simulink model "Model_IPS7"  (R2016a)
settings: Solver=FixedStepAuto  StartTime=0  StopTime=560  FixedStep=1e-5
InitFcn:
  | parametriAM
values from neighbouring files (symbols this model uses):
  Imrn = 7.4    [parametriAM.m]
  Ismax = In*sqrt(2)    [parametriAM.m]
  J = 0.019    [parametriAM.m]    (also in podatki.m = 0.01)
  Ki_Imr = 1000    [parametriAM.m]
  Ki_tok = 5.0    (= 5)    [parametriAM.m]
  Ki_wr = 1000    [parametriAM.m]
  Kp_Imr = 100    [parametriAM.m]
  Kp_tok = 0.05    [parametriAM.m]
  Kp_wr = 50    [parametriAM.m]
  Lm = 0.0493    [parametriAM.m]    (also in podatki.m = 0.2342)
  Lr = 0.05315    [parametriAM.m]    (also in podatki.m = 0.2449)
  Ls = 0.05315    [parametriAM.m]    (also in podatki.m = 0.2449)
  Lst = sigma*Ls    (= 0.00742111947319)    [parametriAM.m]
  naklon = naklon    [parametriAM.m]    (also in staticna_karakteristika.m = 1.0471975512)
  pp = 3    [parametriAM.m]    (also in podatki.m = 2)
  Rs = 0.594    [parametriAM.m]    (also in podatki.m = 3.7)
  sigma = 1 - 1/((1+sigmaR)*(1+sigmaS))    (= 0.13962595434)    [parametriAM.m]
  static_or_dinamic = static_or_dinamic    [parametriAM.m]    (also in potek_toka.m = 0; staticna_karakteristika.m = 5)
  Tr = Lr/Rr    (= 0.0771407837446)    [parametriAM.m]
  Udc = Un*sqrt(2)    [parametriAM.m]
  wb_upper_limit_field_weaking = sqrt((Ls^2+Lst^2)/(2*Lst^2*Ls^2))*Usmax/Ismax    [parametriAM.m]
  wdod = 2000*2*pi/60    (= 209.439510239)    [parametriAM.m]
  wn = Udc/sqrt(Ls^2*(Imrn)^2+Lst^2*(Ismax^2-(Imrn)^2))    [maximalnaelipsa.m]    (also in parametriAM.m = Un/sqrt(Ls^2*(Imrn)^2+Lst^2*(Ismax^2-(Imrn)^2))/pp)
libraries: simulink x25
(part 1 of 2)
settings Model: Creator=Vaje  LastModifiedBy=Mitja1

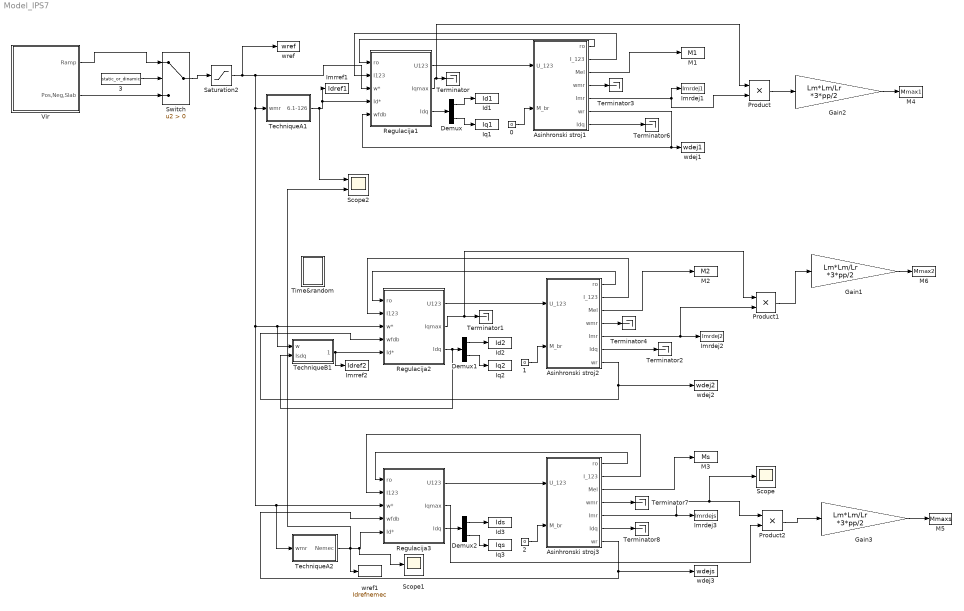
== system Model_IPS7 ==
  0 : Constant  Value=0
  1 : Constant  Value=0
  2 : Constant  Value=0
  3 : Constant  Value=static_or_dinamic
  Asinhronski stroj1 : Subsystem  InitFcn=parametriAM
  Asinhronski stroj2 : Subsystem  InitFcn=parametriAM
  Asinhronski stroj3 : Subsystem  InitFcn=parametriAM
  Demux : Demux  Outputs=2
  Demux1 : Demux  Outputs=2
  Demux2 : Demux  Outputs=2
  Gain1 : Gain  Gain=Lm*Lm/Lr *3*pp/2
  Gain2 : Gain  Gain=Lm*Lm/Lr *3*pp/2
  Gain3 : Gain  Gain=Lm*Lm/Lr *3*pp/2
  Id1 : ToWorkspace  VariableName=Id1  SampleTime=-1
      settings: Decimation=3  Save2DSignal=2-D array (concatenate along first dimension)
  Id2 : ToWorkspace  VariableName=Id2  SampleTime=-1
      settings: Decimation=3  Save2DSignal=2-D array (concatenate along first dimension)
  Id3 : ToWorkspace  VariableName=Ids  SampleTime=-1
      settings: Decimation=3  Save2DSignal=2-D array (concatenate along first dimension)
  Imrdej1 : ToWorkspace  VariableName=Imrdej1  SampleTime=-1
      settings: Decimation=3  Save2DSignal=2-D array (concatenate along first dimension)
  Imrdej2 : ToWorkspace  VariableName=Imrdej2  SampleTime=-1
      settings: Decimation=3  Save2DSignal=2-D array (concatenate along first dimension)
  Imrdej3 : ToWorkspace  VariableName=Imrdejs  SampleTime=-1
      settings: Decimation=3  Save2DSignal=2-D array (concatenate along first dimension)
  Imrref1 : ToWorkspace  VariableName=Idref1  SampleTime=-1
      settings: Decimation=3  Save2DSignal=2-D array (concatenate along first dimension)
  Imrref2 : ToWorkspace  VariableName=Idref2  SampleTime=-1
      settings: Decimation=3  Save2DSignal=2-D array (concatenate along first dimension)
  Iq1 : ToWorkspace  VariableName=Iq1  SampleTime=-1
      settings: Decimation=3  Save2DSignal=2-D array (concatenate along first dimension)
  Iq2 : ToWorkspace  VariableName=Iq2  SampleTime=-1
      settings: Decimation=3  Save2DSignal=2-D array (concatenate along first dimension)
  Iq3 : ToWorkspace  VariableName=Iqs  SampleTime=-1
      settings: Decimation=3  Save2DSignal=2-D array (concatenate along first dimension)
  M1 : ToWorkspace  VariableName=M1  SampleTime=-1
      settings: Decimation=3  Save2DSignal=2-D array (concatenate along first dimension)
  M2 : ToWorkspace  VariableName=M2  SampleTime=-1
      settings: Decimation=3  Save2DSignal=2-D array (concatenate along first dimension)
  M3 : ToWorkspace  VariableName=Ms  SampleTime=-1
      settings: Decimation=3  Save2DSignal=2-D array (concatenate along first dimension)
  M4 : ToWorkspace  VariableName=Mmax1  SampleTime=-1
      settings: Decimation=3  Save2DSignal=2-D array (concatenate along first dimension)
  M5 : ToWorkspace  VariableName=Mmaxs  SampleTime=-1
      settings: Decimation=3  Save2DSignal=2-D array (concatenate along first dimension)
  M6 : ToWorkspace  VariableName=Mmax2  SampleTime=-1
      settings: Decimation=3  Save2DSignal=2-D array (concatenate along first dimension)
  Product : Product
  Product1 : Product
  Product2 : Product
  Regulacija1 : Subsystem
  Regulacija2 : Subsystem
  Regulacija3 : Subsystem
  Saturation2 : Saturate  UpperLimit=wb_upper_limit_field_weaking  LowerLimit=-wb_upper_limit_field_weaking
  Scope : Scope
  Scope1 : Scope
  Scope2 : Scope  NumInputPorts=2
  Switch : Switch  Criteria=u2 > Threshold
  TechniqueA1 : Subsystem
  TechniqueA2 : Subsystem
  TechniqueB1 : Subsystem
  Terminator{,1..4,6..8} (8 alike) : Terminator
  Time&random : Subsystem
  Vir : Subsystem
  wdej1 : ToWorkspace  VariableName=wdej1  SampleTime=-1
      settings: Decimation=3  Save2DSignal=2-D array (concatenate along first dimension)
  wdej2 : ToWorkspace  VariableName=wdej2  SampleTime=-1
      settings: Decimation=3  Save2DSignal=2-D array (concatenate along first dimension)
  wdej3 : ToWorkspace  VariableName=wdejs  SampleTime=-1
      settings: Decimation=3  Save2DSignal=2-D array (concatenate along first dimension)
  wref : ToWorkspace  VariableName=wref  SampleTime=-1
      settings: Decimation=3  Save2DSignal=2-D array (concatenate along first dimension)
  wref1 : ToWorkspace  VariableName=Idrefnemec  SampleTime=-1
      settings: Decimation=3  Save2DSignal=2-D array (concatenate along first dimension)
  wires:
  Vir/2(Pos,Neg,Slab) -> Switch/3
  TechniqueA1/1(6.1-126) -> Scope2/1, Regulacija1/4(Id*), Imrref1/1
  Asinhronski stroj1/1(ro) -> Regulacija1/1(ro)
  Asinhronski stroj1/2(I_123) -> Regulacija1/2(I123)
  Regulacija1/1(U123) -> Asinhronski stroj1/1(U_123)
  Asinhronski stroj1/6(wr) -> Regulacija1/5(wfdb), wdej1/1
  Switch/1 -> Saturation2/1
  Asinhronski stroj2/1(ro) -> Regulacija2/1(ro)
  Asinhronski stroj2/2(I_123) -> Regulacija2/2(I123)
  Regulacija2/1(U123) -> Asinhronski stroj2/1(U_123)
  Saturation2/1 -> Regulacija1/3(w*), TechniqueA1/1(wmr), TechniqueA2/1(wmr), Regulacija3/3(w*), TechniqueB1/1(w), Regulacija2/3(w*), wref/1
  Regulacija2/3(Idq) -> TechniqueB1/2(Isdq), Demux1/1
  TechniqueB1/1(6.1-135) -> Regulacija2/5(Id*), Imrref2/1
  Asinhronski stroj1/5(Imr) -> Product/2, Imrdej1/1
  Asinhronski stroj2/5(Imr) -> Product1/2, Imrdej2/1
  Asinhronski stroj1/3(Mel) -> M1/1
  Asinhronski stroj2/3(Mel) -> M2/1
  Demux/2 -> Iq1/1
  Demux/1 -> Id1/1
  Demux1/1 -> Id2/1
  Demux1/2 -> Iq2/1
  Regulacija1/3(Idq) -> Demux/1
  Regulacija1/2(Iqmax) -> Product/1, Terminator/1
  Regulacija2/2(Iqmax) -> Product1/1, Terminator1/1
  Asinhronski stroj2/6(Idq) -> Terminator2/1
  0/1 -> Asinhronski stroj1/2(M_br)
  1/1 -> Asinhronski stroj2/2(M_br)
  Asinhronski stroj1/7(Idq) -> Terminator6/1
  Asinhronski stroj1/4(wmr) -> Terminator3/1
  Asinhronski stroj2/4(wmr) -> Terminator4/1
  Regulacija3/1(U123) -> Asinhronski stroj3/1(U_123)
  Regulacija3/3(Idq) -> Demux2/1
  Demux2/1 -> Id3/1
  Demux2/2 -> Iq3/1
  Regulacija3/2(Iqmax) -> Product2/2
  2/1 -> Asinhronski stroj3/2(M_br)
  Asinhronski stroj3/1(ro) -> Regulacija3/1(ro)
  Asinhronski stroj3/2(I_123) -> Regulacija3/2(I123)
  Asinhronski stroj3/5(Imr) -> Scope/1, Product2/1, Imrdej3/1
  Asinhronski stroj3/3(Mel) -> M3/1
  Asinhronski stroj3/4(wmr) -> Terminator7/1
  Asinhronski stroj3/6(Idq) -> Terminator8/1
  Product/1 -> Gain2/1
  Product1/1 -> Gain1/1
  Product2/1 -> Gain3/1
  Gain2/1 -> M4/1
  Gain3/1 -> M5/1
  Gain1/1 -> M6/1
  3/1 -> Switch/2
  Asinhronski stroj3/7(wr) -> wdej3/1, Regulacija3/4(wfdb)
  Asinhronski stroj2/7(wr) -> Regulacija2/4(wfdb), wdej2/1
  Vir/1(Ramp) -> Switch/1
  TechniqueA2/1(Nemec) -> Scope2/2, wref1/1, Scope1/1, Regulacija3/5(Id*)

== system Model_IPS7/Asinhronski stroj1 ==
  U_123 : Inport
  M_br : Inport  Port=2
  Clarke : Subsystem
  Inverzni Clarke : Subsystem
  Inverzni Park : Subsystem
  Mehanika : Subsystem
  Park : Subsystem
  napetostni dq model : Subsystem
  ro : Outport
  I_123 : Outport  Port=2
  Mel : Outport  Port=3
  wmr : Outport  Port=4
  Imr : Outport  Port=5
  wr : Outport  Port=6
  Idq : Outport  Port=7
  wires:
  Inverzni Park/1(I_ab) -> Inverzni Clarke/1(I_ab)
  Clarke/1(U_ab) -> Park/1(U_ab)
  Mehanika/1(wr) -> napetostni dq model/2(wr), wr/1
  M_br/1 -> Mehanika/1(M_br)
  napetostni dq model/1(Mel) -> Mel/1, Mehanika/2(M_el)
  Inverzni Clarke/1(I_123) -> I_123/1
  napetostni dq model/4(wmr) -> wmr/1
  napetostni dq model/3(Imr) -> Imr/1
  U_123/1 -> Clarke/1(U_123)
  napetostni dq model/2(Is_dq) -> Idq/1, Inverzni Park/1(I_dq)
  napetostni dq model/5(ro) -> ro/1, Park/2(kot), Inverzni Park/2(kot)
  Park/1(U_dq) -> napetostni dq model/1(Us_dq)

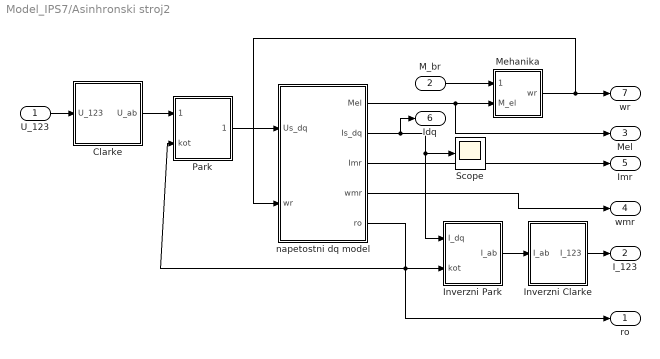
== system Model_IPS7/Asinhronski stroj2 ==
  U_123 : Inport
  M_br : Inport  Port=2
  Clarke : Subsystem
  Inverzni Clarke : Subsystem
  Inverzni Park : Subsystem
  Mehanika : Subsystem
  Park : Subsystem
  Scope : Scope
  napetostni dq model : Subsystem
  ro : Outport
  I_123 : Outport  Port=2
  Mel : Outport  Port=3
  wmr : Outport  Port=4
  Imr : Outport  Port=5
  Idq : Outport  Port=6
  wr : Outport  Port=7
  wires:
  Inverzni Park/1(I_ab) -> Inverzni Clarke/1(I_ab)
  Clarke/1(U_ab) -> Park/1(U_ab)
  Mehanika/1(wr) -> napetostni dq model/2(wr), wr/1
  M_br/1 -> Mehanika/1(M_br)
  napetostni dq model/1(Mel) -> Mel/1, Mehanika/2(M_el)
  Inverzni Clarke/1(I_123) -> I_123/1
  napetostni dq model/4(wmr) -> wmr/1
  napetostni dq model/3(Imr) -> Imr/1
  U_123/1 -> Clarke/1(U_123)
  napetostni dq model/2(Is_dq) -> Idq/1, Scope/1, Inverzni Park/1(I_dq)
  napetostni dq model/5(ro) -> ro/1, Park/2(kot), Inverzni Park/2(kot)
  Park/1(U_dq) -> napetostni dq model/1(Us_dq)

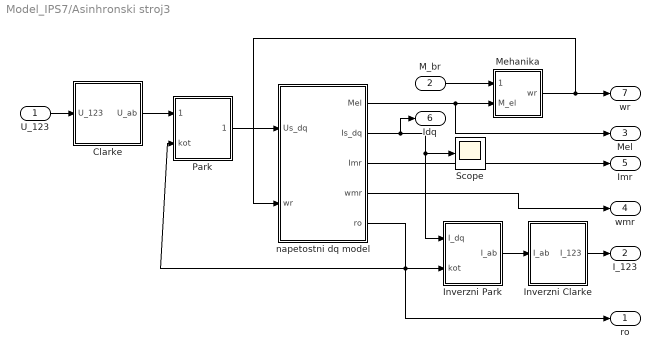
== system Model_IPS7/Asinhronski stroj3 ==
  U_123 : Inport
  M_br : Inport  Port=2
  Clarke : Subsystem
  Inverzni Clarke : Subsystem
  Inverzni Park : Subsystem
  Mehanika : Subsystem
  Park : Subsystem
  Scope : Scope
  napetostni dq model : Subsystem
  ro : Outport
  I_123 : Outport  Port=2
  Mel : Outport  Port=3
  wmr : Outport  Port=4
  Imr : Outport  Port=5
  Idq : Outport  Port=6
  wr : Outport  Port=7
  wires:
  Park/1(U_dq) -> napetostni dq model/1(Us_dq)
  napetostni dq model/5(ro) -> Inverzni Park/2(kot), Park/2(kot), ro/1
  napetostni dq model/2(Is_dq) -> Inverzni Park/1(I_dq), Scope/1, Idq/1
  U_123/1 -> Clarke/1(U_123)
  napetostni dq model/3(Imr) -> Imr/1
  napetostni dq model/4(wmr) -> wmr/1
  Inverzni Clarke/1(I_123) -> I_123/1
  napetostni dq model/1(Mel) -> Mehanika/2(M_el), Mel/1
  M_br/1 -> Mehanika/1(M_br)
  Mehanika/1(wr) -> wr/1, napetostni dq model/2(wr)
  Clarke/1(U_ab) -> Park/1(U_ab)
  Inverzni Park/1(I_ab) -> Inverzni Clarke/1(I_ab)

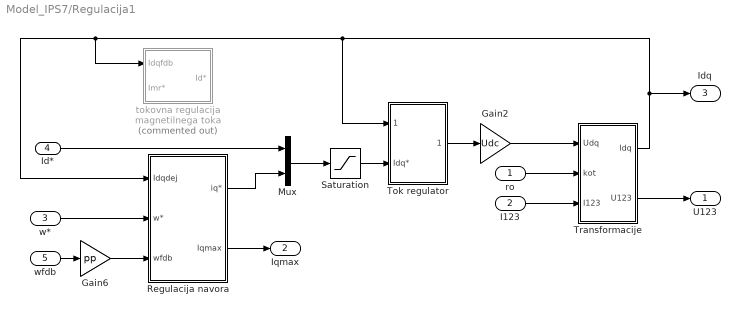
== system Model_IPS7/Regulacija1 ==
  ro : Inport
  I123 : Inport  Port=2
  w* : Inport  Port=3
  Id* : Inport  Port=4
  wfdb : Inport  Port=5
  Gain2 : Gain  Gain=Udc
  Gain6 : Gain  Gain=pp
  Mux : Mux  Inputs=2
  Regulacija navora : Subsystem
  Saturation : Saturate  UpperLimit=Ismax  LowerLimit=-Ismax
  Tok regulator : Subsystem
  Transformacije : Subsystem
  tokovna regulacija magnetilnega toka : Subsystem  Commented=on
  U123 : Outport
  Iqmax : Outport  Port=2
  Idq : Outport  Port=3
  wires:
  w*/1 -> Regulacija navora/2(w*)
  Transformacije/1(Idq) -> Idq/1, Tok regulator/1(Idqdej), tokovna regulacija magnetilnega toka/1(Idqfdb), Regulacija navora/1(Idqdej)
  ro/1 -> Transformacije/2(kot)
  I123/1 -> Transformacije/3(I123)
  Gain2/1 -> Transformacije/1(Udq)
  wfdb/1 -> Gain6/1
  Mux/1 -> Saturation/1
  Tok regulator/1(Udq*) -> Gain2/1
  Regulacija navora/1(iq*) -> Mux/2
  Transformacije/2(U123) -> U123/1
  Regulacija navora/2(Iqmax) -> Iqmax/1
  Gain6/1 -> Regulacija navora/3(wfdb)
  Saturation/1 -> Tok regulator/2(Idq*)
  Id*/1 -> Mux/1

== system Model_IPS7/Regulacija2 ==
  ro : Inport
  I123 : Inport  Port=2
  w* : Inport  Port=3
  wfdb : Inport  Port=4
  Id* : Inport  Port=5
  Gain2 : Gain  Gain=Udc
  Gain6 : Gain  Gain=pp
  Mux : Mux  Inputs=2
  Regulacija navora : Subsystem
  Tok regulator : Subsystem
  Transformacije : Subsystem
  tokovna regulacija magnetilnega toka : Subsystem  Commented=on
  U123 : Outport
  Iqmax : Outport  Port=2
  Idq : Outport  Port=3
  wires:
  Id*/1 -> Mux/1
  w*/1 -> Regulacija navora/2(w*)
  Transformacije/1(Idq) -> Tok regulator/1(Idqdej), Regulacija navora/1(Idqdej), tokovna regulacija magnetilnega toka/1(Idqfdb), Idq/1
  ro/1 -> Transformacije/2(kot)
  I123/1 -> Transformacije/3(I123)
  Gain2/1 -> Transformacije/1(Udq)
  wfdb/1 -> Gain6/1
  Mux/1 -> Tok regulator/2(Idq*)
  Tok regulator/1(Udq*) -> Gain2/1
  Regulacija navora/1(Iq*) -> Mux/2
  Transformacije/2(U123) -> U123/1
  Regulacija navora/2(Iqmax) -> Iqmax/1
  Gain6/1 -> Regulacija navora/3(wfdb)

== system Model_IPS7/Regulacija3 ==
  ro : Inport
  I123 : Inport  Port=2
  w* : Inport  Port=3
  wfdb : Inport  Port=4
  Id* : Inport  Port=5
  Gain2 : Gain  Gain=Udc
  Gain6 : Gain  Gain=pp
  Mux : Mux  Inputs=2
  Regulacija navora : Subsystem
  Tok regulator : Subsystem
  Transformacije : Subsystem
  tokovna regulacija magnetilnega toka : Subsystem
  U123 : Outport
  Iqmax : Outport  Port=2
  Idq : Outport  Port=3
  wires:
  Gain6/1 -> Regulacija navora/3(wfdb)
  Regulacija navora/2(Iqmax) -> Iqmax/1
  Transformacije/2(U123) -> U123/1
  Regulacija navora/1(Iq*) -> Mux/2
  Tok regulator/1(Udq*) -> Gain2/1
  Mux/1 -> Tok regulator/2(Idq*)
  wfdb/1 -> Gain6/1
  Gain2/1 -> Transformacije/1(Udq)
  I123/1 -> Transformacije/3(I123)
  ro/1 -> Transformacije/2(kot)
  Transformacije/1(Idq) -> Idq/1, tokovna regulacija magnetilnega toka/1(Idqfdb), Regulacija navora/1(Idqdej), Tok regulator/1(Idqdej)
  w*/1 -> Regulacija navora/2(w*)
  tokovna regulacija magnetilnega toka/1(Id*) -> Mux/1
  Id*/1 -> tokovna regulacija magnetilnega toka/2(Imr*)

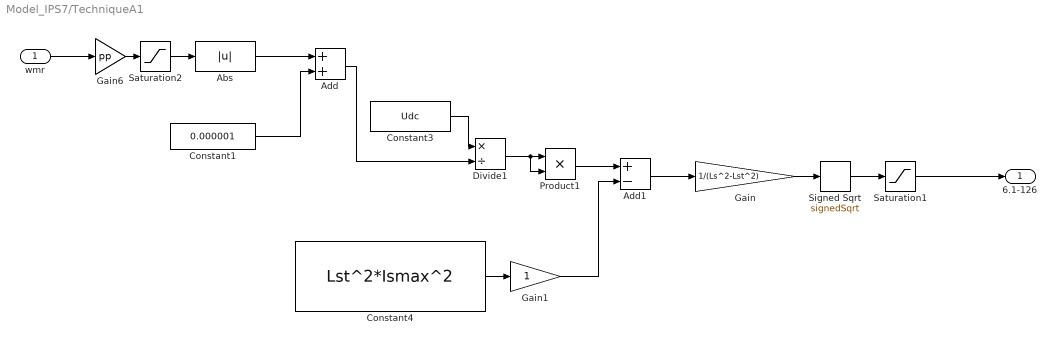
== system Model_IPS7/TechniqueA1 ==
  wmr : Inport
  Abs : Abs
  Add : Sum
  Add1 : Sum  Inputs=+-
  Constant1 : Constant  Value=0.000001
  Constant3 : Constant  Value=Udc
  Constant4 : Constant  Value=Lst^2*Ismax^2
  Divide1 : Product  Inputs=*/
  Gain : Gain  Gain=1/(Ls^2-Lst^2)
  Gain1 : Gain
  Gain6 : Gain  Gain=pp
  Product1 : Product
  Saturation1 : Saturate  UpperLimit=+Imrn*sqrt(2)  LowerLimit=-Imrn*sqrt(2)
  Saturation2 : Saturate  UpperLimit=wb_upper_limit_field_weaking  LowerLimit=-wb_upper_limit_field_weaking
  Signed Sqrt : Sqrt  Operator=signedSqrt  SaturateOnIntegerOverflow=on
  6.1-126 : Outport
  wires:
  Add/1 -> Divide1/2
  Abs/1 -> Add/1
  Constant1/1 -> Add/2
  Constant3/1 -> Divide1/1
  Divide1/1 -> Product1/2, Product1/1
  Product1/1 -> Add1/1
  Saturation1/1 -> 6.1-126/1
  Add1/1 -> Gain/1
  Gain/1 -> Signed Sqrt/1
  Signed Sqrt/1 -> Saturation1/1
  Saturation2/1 -> Abs/1
  Constant4/1 -> Gain1/1
  Gain1/1 -> Add1/2
  Gain6/1 -> Saturation2/1
  wmr/1 -> Gain6/1

== system Model_IPS7/TechniqueA2 ==
  wmr : Inport
  Abs : Abs
  Add : Sum
  Constant : Constant  Value=wn
  Constant1 : Constant  Value=0.000001
  Constant2 : Constant  Value=Imrn*sqrt(2)
  Divide : Product  Inputs=*/
  Product : Product
  Saturation : Saturate  UpperLimit=+Imrn*sqrt(2)  LowerLimit=-Imrn*sqrt(2)
  Saturation2 : Saturate  UpperLimit=wb_upper_limit_field_weaking  LowerLimit=-wb_upper_limit_field_weaking
  Nemec : Outport
  wires:
  Saturation2/1 -> Abs/1
  Saturation/1 -> Nemec/1
  Constant1/1 -> Add/2
  Abs/1 -> Add/1
  Add/1 -> Divide/2
  Constant/1 -> Divide/1
  Product/1 -> Saturation/1
  Divide/1 -> Product/2
  Constant2/1 -> Product/1
  wmr/1 -> Saturation2/1

== system Model_IPS7/TechniqueB1 ==
  w : Inport
  Isdq : Inport  Port=2
  Add4 : Sum
  Const c : Subsystem
  Deljeno imenovalec 6.1-135 : Gain  Gain=1/(Ls^2-Lst^2)
  Demux : Demux  Outputs=2
  Gain4 : Gain  Gain=-Ls
  Gain6 : Gain  Gain=pp
  Korenski del : Subsystem
  Saturation : Saturate  UpperLimit=+Imrn*sqrt(2)  LowerLimit=-Imrn*sqrt(2)
  Terminator : Terminator
  6.1-135 : Outport
  wires:
  Demux/1 -> Const c/1(Id)
  Demux/2 -> Terminator/1
  Saturation/1 -> 6.1-135/1
  Const c/1(c) -> Korenski del/1(c), Gain4/1
  Gain4/1 -> Add4/1
  Add4/1 -> Deljeno imenovalec 6.1-135/1
  Deljeno imenovalec 6.1-135/1 -> Saturation/1
  Isdq/1 -> Demux/1
  Korenski del/1(korenjen del) -> Add4/2
  w/1 -> Gain6/1
  Gain6/1 -> Korenski del/2(w)

== system Model_IPS7/Time&random ==
  99% max navora : Subsystem  Commented=on
  Mux1 : Mux  Commented=on  Inputs=2
  Ramp : simulink/Sources/Ramp  slope=1  start=0  X0=0
  To Workspace3 : ToWorkspace  VariableName=time  SampleTime=-1
      settings: Decimation=3  Save2DSignal=2-D array (concatenate along first dimension)
  wires:
  Ramp/1 -> To Workspace3/1

== system Model_IPS7/Vir ==
  Add1 : Sum
  Rampa : simulink/Sources/Ramp  slope=naklon  start=0.3  X0=0
  Step : Step  Time=0.1  After=2000*2*pi/60  SampleTime=0
  Step1 : Step  Time=0.7  After=2000*pi/30  SampleTime=0
  Step2 : Step  Commented=on  Time=2  After=2000*2*pi/60  SampleTime=0
  Step3 : Step  Commented=on  Time=3  After=2000*2*pi/60  SampleTime=0
  Step4 : Step  Commented=on  Time=8  After=wdod  SampleTime=0
  Step5 : Step  Commented=on  Time=9  After=wdod  SampleTime=0
  Ramp : Outport
  Pos,Neg,Slab : Outport  Port=2
  wires:
  Add1/1 -> Pos,Neg,Slab/1
  Step/1 -> Add1/1
  Rampa/1 -> Ramp/1
  Step1/1 -> Add1/2

== system Model_IPS7/Asinhronski stroj1/Clarke ==
  U_123 : Inport
  ABC_ab1 : Subsystem
  Demux : Demux  Outputs=3
  Mux : Mux  Inputs=2
  U_ab : Outport
  wires:
  Mux/1 -> U_ab/1
  ABC_ab1/2(beta) -> Mux/2
  ABC_ab1/1(alfa) -> Mux/1
  Demux/3 -> ABC_ab1/3(C)
  Demux/2 -> ABC_ab1/2(B)
  Demux/1 -> ABC_ab1/1(A)
  U_123/1 -> Demux/1

== system Model_IPS7/Asinhronski stroj1/Inverzni Clarke ==
  I_ab : Inport
  Demux : Demux  Outputs=2
  Mux : Mux  Inputs=3
  ab_ABC : Subsystem
  I_123 : Outport
  wires:
  ab_ABC/3(C) -> Mux/3
  ab_ABC/2(B) -> Mux/2
  ab_ABC/1(A) -> Mux/1
  Demux/2 -> ab_ABC/2(beta)
  Demux/1 -> ab_ABC/1(alfa)
  I_ab/1 -> Demux/1
  Mux/1 -> I_123/1

== system Model_IPS7/Asinhronski stroj1/Inverzni Park ==
  I_dq : Inport
  kot : Inport  Port=2
  Demux : Demux  Outputs=2
  Mux : Mux  Inputs=2
  "Sum1 " : Sum  Inputs=+-  SaturateOnIntegerOverflow=on  InputSameDT=on  OutDataTypeStr=Inherit: Same as first input
  Sum2 : Sum  SaturateOnIntegerOverflow=on  InputSameDT=on  OutDataTypeStr=Inherit: Same as first input
  cos : Fcn  Expr=cos(u)
  sin : Fcn  Expr=sin(u)
  x_d*cos : Product  SaturateOnIntegerOverflow=on  RndMeth=Zero  InputSameDT=on  OutDataTypeStr=Inherit: Same as first input
  x_d*sin : Product  SaturateOnIntegerOverflow=on  RndMeth=Zero  InputSameDT=on  OutDataTypeStr=Inherit: Same as first input
  x_q*cos : Product  SaturateOnIntegerOverflow=on  RndMeth=Zero  InputSameDT=on  OutDataTypeStr=Inherit: Same as first input
  "x_q*sin " : Product  SaturateOnIntegerOverflow=on  RndMeth=Zero  InputSameDT=on  OutDataTypeStr=Inherit: Same as first input
  I_ab : Outport
  wires:
  Mux/1 -> I_ab/1
  I_dq/1 -> Demux/1
  Demux/1 -> x_d*sin/1, x_d*cos/1
  Demux/2 -> "x_q*sin "/1, x_q*cos/1
  cos/1 -> x_q*cos/2, x_d*cos/2
  sin/1 -> "x_q*sin "/2, x_d*sin/2
  x_d*cos/1 -> "Sum1 "/1
  "x_q*sin "/1 -> "Sum1 "/2
  x_q*cos/1 -> Sum2/2
  x_d*sin/1 -> Sum2/1
  "Sum1 "/1 -> Mux/1
  Sum2/1 -> Mux/2
  kot/1 -> cos/1, sin/1

== system Model_IPS7/Asinhronski stroj1/Mehanika ==
  M_br : Inport
  M_el : Inport  Port=2
  Sum : Sum  Inputs=+-
  eq 2.19 : Subsystem
  wr : Outport
  wires:
  M_br/1 -> Sum/2
  Sum/1 -> eq 2.19/1(M)
  M_el/1 -> Sum/1
  eq 2.19/1(wr) -> wr/1

== system Model_IPS7/Asinhronski stroj1/Park ==
  U_ab : Inport
  kot : Inport  Port=2
  Demux : Demux  Outputs=2
  Mux : Mux  Inputs=2
  "Sum1 " : Sum  SaturateOnIntegerOverflow=on  InputSameDT=on  OutDataTypeStr=Inherit: Same as first input
  Sum2 : Sum  Inputs=-+  SaturateOnIntegerOverflow=on  InputSameDT=on  OutDataTypeStr=Inherit: Same as first input
  cos : Fcn  Expr=cos(u)
  sin : Fcn  Expr=sin(u)
  x_a*cos : Product  SaturateOnIntegerOverflow=on  RndMeth=Zero  InputSameDT=on  OutDataTypeStr=Inherit: Same as first input
  x_a*sin : Product  SaturateOnIntegerOverflow=on  RndMeth=Zero  InputSameDT=on  OutDataTypeStr=Inherit: Same as first input
  x_b*cos : Product  SaturateOnIntegerOverflow=on  RndMeth=Zero  InputSameDT=on  OutDataTypeStr=Inherit: Same as first input
  "x_b*sin " : Product  SaturateOnIntegerOverflow=on  RndMeth=Zero  InputSameDT=on  OutDataTypeStr=Inherit: Same as first input
  U_dq : Outport
  wires:
  Mux/1 -> U_dq/1
  U_ab/1 -> Demux/1
  Demux/1 -> x_a*sin/1, x_a*cos/1
  Demux/2 -> "x_b*sin "/1, x_b*cos/1
  cos/1 -> x_b*cos/2, x_a*cos/2
  sin/1 -> "x_b*sin "/2, x_a*sin/2
  x_a*cos/1 -> "Sum1 "/1
  "x_b*sin "/1 -> "Sum1 "/2
  x_b*cos/1 -> Sum2/2
  x_a*sin/1 -> Sum2/1
  "Sum1 "/1 -> Mux/1
  Sum2/1 -> Mux/2
  kot/1 -> cos/1, sin/1

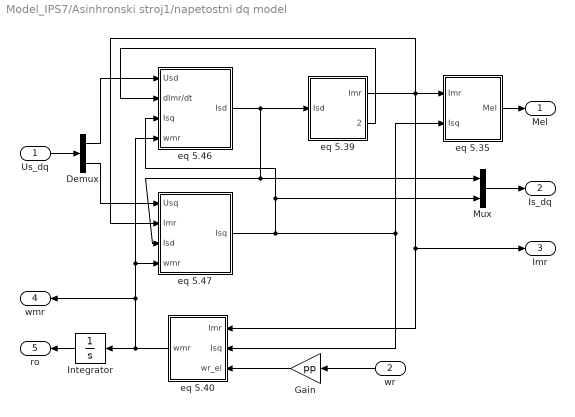
== system Model_IPS7/Asinhronski stroj1/napetostni dq model ==
  Us_dq : Inport
  wr : Inport  Port=2
  Demux : Demux  Outputs=2
  Gain : Gain  Gain=pp
  Integrator : Integrator
  Mux : Mux  Inputs=2
  eq 5.35 : Subsystem
  eq 5.39 : Subsystem
  eq 5.40 : Subsystem
  eq 5.46 : Subsystem
  eq 5.47 : Subsystem
  Mel : Outport
  Is_dq : Outport  Port=2
  Imr : Outport  Port=3
  wmr : Outport  Port=4
  ro : Outport  Port=5
  wires:
  Gain/1 -> eq 5.40/3(wr_el)
  Mux/1 -> Is_dq/1
  Demux/2 -> eq 5.47/1(Usq)
  Demux/1 -> eq 5.46/1(Usd)
  Us_dq/1 -> Demux/1
  wr/1 -> Gain/1
  Integrator/1 -> ro/1
  eq 5.35/1(Mel) -> Mel/1
  eq 5.40/1(wmr) -> Integrator/1, wmr/1, eq 5.46/4(wmr), eq 5.47/4(wmr)
  eq 5.47/1(Isq) -> Mux/2, eq 5.46/3(Isq), eq 5.40/2(Isq), eq 5.35/2(Isq)
  eq 5.39/1(Imr) -> eq 5.47/2(Imr), Imr/1, eq 5.40/1(Imr), eq 5.35/1(Imr)
  eq 5.39/2(dImr/dt) -> eq 5.46/2(dImr/dt)
  eq 5.46/1(Isd) -> Mux/1, eq 5.47/3(Isd), eq 5.39/1(Isd)

== system Model_IPS7/Asinhronski stroj2/Clarke ==
  U_123 : Inport
  ABC_ab1 : Subsystem
  Demux : Demux  Outputs=3
  Mux : Mux  Inputs=2
  U_ab : Outport
  wires:
  Mux/1 -> U_ab/1
  ABC_ab1/2(beta) -> Mux/2
  ABC_ab1/1(alfa) -> Mux/1
  Demux/3 -> ABC_ab1/3(C)
  Demux/2 -> ABC_ab1/2(B)
  Demux/1 -> ABC_ab1/1(A)
  U_123/1 -> Demux/1

== system Model_IPS7/Asinhronski stroj2/Inverzni Clarke ==
  I_ab : Inport
  Demux : Demux  Outputs=2
  Mux : Mux  Inputs=3
  ab_ABC : Subsystem
  I_123 : Outport
  wires:
  ab_ABC/3(C) -> Mux/3
  ab_ABC/2(B) -> Mux/2
  ab_ABC/1(A) -> Mux/1
  Demux/2 -> ab_ABC/2(beta)
  Demux/1 -> ab_ABC/1(alfa)
  I_ab/1 -> Demux/1
  Mux/1 -> I_123/1

== system Model_IPS7/Asinhronski stroj2/Inverzni Park ==
  I_dq : Inport
  kot : Inport  Port=2
  Demux : Demux  Outputs=2
  Mux : Mux  Inputs=2
  "Sum1 " : Sum  Inputs=+-  SaturateOnIntegerOverflow=on  InputSameDT=on  OutDataTypeStr=Inherit: Same as first input
  Sum2 : Sum  SaturateOnIntegerOverflow=on  InputSameDT=on  OutDataTypeStr=Inherit: Same as first input
  cos : Fcn  Expr=cos(u)
  sin : Fcn  Expr=sin(u)
  x_d*cos : Product  SaturateOnIntegerOverflow=on  RndMeth=Zero  InputSameDT=on  OutDataTypeStr=Inherit: Same as first input
  x_d*sin : Product  SaturateOnIntegerOverflow=on  RndMeth=Zero  InputSameDT=on  OutDataTypeStr=Inherit: Same as first input
  x_q*cos : Product  SaturateOnIntegerOverflow=on  RndMeth=Zero  InputSameDT=on  OutDataTypeStr=Inherit: Same as first input
  "x_q*sin " : Product  SaturateOnIntegerOverflow=on  RndMeth=Zero  InputSameDT=on  OutDataTypeStr=Inherit: Same as first input
  I_ab : Outport
  wires:
  Mux/1 -> I_ab/1
  I_dq/1 -> Demux/1
  Demux/1 -> x_d*sin/1, x_d*cos/1
  Demux/2 -> "x_q*sin "/1, x_q*cos/1
  cos/1 -> x_q*cos/2, x_d*cos/2
  sin/1 -> "x_q*sin "/2, x_d*sin/2
  x_d*cos/1 -> "Sum1 "/1
  "x_q*sin "/1 -> "Sum1 "/2
  x_q*cos/1 -> Sum2/2
  x_d*sin/1 -> Sum2/1
  "Sum1 "/1 -> Mux/1
  Sum2/1 -> Mux/2
  kot/1 -> cos/1, sin/1

== system Model_IPS7/Asinhronski stroj2/Mehanika ==
  M_br : Inport
  M_el : Inport  Port=2
  Sum : Sum  Inputs=+-
  eq 2.19 : Subsystem
  wr : Outport
  wires:
  M_br/1 -> Sum/2
  Sum/1 -> eq 2.19/1(M)
  M_el/1 -> Sum/1
  eq 2.19/1(wr) -> wr/1

== system Model_IPS7/Asinhronski stroj2/Park ==
  U_ab : Inport
  kot : Inport  Port=2
  Demux : Demux  Outputs=2
  Mux : Mux  Inputs=2
  "Sum1 " : Sum  SaturateOnIntegerOverflow=on  InputSameDT=on  OutDataTypeStr=Inherit: Same as first input
  Sum2 : Sum  Inputs=-+  SaturateOnIntegerOverflow=on  InputSameDT=on  OutDataTypeStr=Inherit: Same as first input
  cos : Fcn  Expr=cos(u)
  sin : Fcn  Expr=sin(u)
  x_a*cos : Product  SaturateOnIntegerOverflow=on  RndMeth=Zero  InputSameDT=on  OutDataTypeStr=Inherit: Same as first input
  x_a*sin : Product  SaturateOnIntegerOverflow=on  RndMeth=Zero  InputSameDT=on  OutDataTypeStr=Inherit: Same as first input
  x_b*cos : Product  SaturateOnIntegerOverflow=on  RndMeth=Zero  InputSameDT=on  OutDataTypeStr=Inherit: Same as first input
  "x_b*sin " : Product  SaturateOnIntegerOverflow=on  RndMeth=Zero  InputSameDT=on  OutDataTypeStr=Inherit: Same as first input
  U_dq : Outport
  wires:
  Mux/1 -> U_dq/1
  U_ab/1 -> Demux/1
  Demux/1 -> x_a*sin/1, x_a*cos/1
  Demux/2 -> "x_b*sin "/1, x_b*cos/1
  cos/1 -> x_b*cos/2, x_a*cos/2
  sin/1 -> "x_b*sin "/2, x_a*sin/2
  x_a*cos/1 -> "Sum1 "/1
  "x_b*sin "/1 -> "Sum1 "/2
  x_b*cos/1 -> Sum2/2
  x_a*sin/1 -> Sum2/1
  "Sum1 "/1 -> Mux/1
  Sum2/1 -> Mux/2
  kot/1 -> cos/1, sin/1

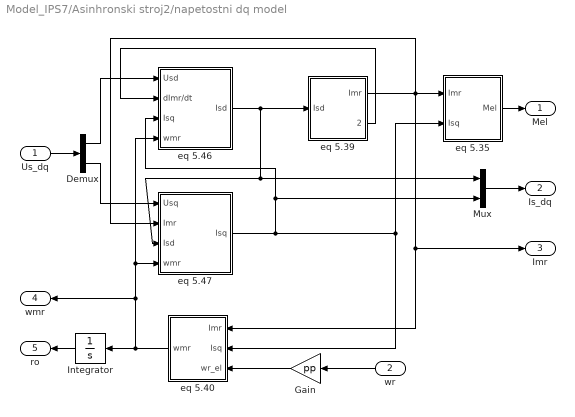
== system Model_IPS7/Asinhronski stroj2/napetostni dq model ==
  Us_dq : Inport
  wr : Inport  Port=2
  Demux : Demux  Outputs=2
  Gain : Gain  Gain=pp
  Integrator : Integrator
  Mux : Mux  Inputs=2
  eq 5.35 : Subsystem
  eq 5.39 : Subsystem
  eq 5.40 : Subsystem
  eq 5.46 : Subsystem
  eq 5.47 : Subsystem
  Mel : Outport
  Is_dq : Outport  Port=2
  Imr : Outport  Port=3
  wmr : Outport  Port=4
  ro : Outport  Port=5
  wires:
  Gain/1 -> eq 5.40/3(wr_el)
  Mux/1 -> Is_dq/1
  Demux/2 -> eq 5.47/1(Usq)
  Demux/1 -> eq 5.46/1(Usd)
  Us_dq/1 -> Demux/1
  wr/1 -> Gain/1
  Integrator/1 -> ro/1
  eq 5.35/1(Mel) -> Mel/1
  eq 5.40/1(wmr) -> Integrator/1, wmr/1, eq 5.46/4(wmr), eq 5.47/4(wmr)
  eq 5.47/1(Isq) -> Mux/2, eq 5.46/3(Isq), eq 5.40/2(Isq), eq 5.35/2(Isq)
  eq 5.39/1(Imr) -> eq 5.47/2(Imr), Imr/1, eq 5.40/1(Imr), eq 5.35/1(Imr)
  eq 5.39/2(dImr/dt) -> eq 5.46/2(dImr/dt)
  eq 5.46/1(Isd) -> Mux/1, eq 5.47/3(Isd), eq 5.39/1(Isd)

== system Model_IPS7/Asinhronski stroj3/Clarke ==
  U_123 : Inport
  ABC_ab1 : Subsystem
  Demux : Demux  Outputs=3
  Mux : Mux  Inputs=2
  U_ab : Outport
  wires:
  U_123/1 -> Demux/1
  Demux/1 -> ABC_ab1/1(A)
  Demux/2 -> ABC_ab1/2(B)
  Demux/3 -> ABC_ab1/3(C)
  ABC_ab1/1(alfa) -> Mux/1
  ABC_ab1/2(beta) -> Mux/2
  Mux/1 -> U_ab/1

== system Model_IPS7/Asinhronski stroj3/Inverzni Clarke ==
  I_ab : Inport
  Demux : Demux  Outputs=2
  Mux : Mux  Inputs=3
  ab_ABC : Subsystem
  I_123 : Outport
  wires:
  Mux/1 -> I_123/1
  I_ab/1 -> Demux/1
  Demux/1 -> ab_ABC/1(alfa)
  Demux/2 -> ab_ABC/2(beta)
  ab_ABC/1(A) -> Mux/1
  ab_ABC/2(B) -> Mux/2
  ab_ABC/3(C) -> Mux/3

== system Model_IPS7/Asinhronski stroj3/Inverzni Park ==
  I_dq : Inport
  kot : Inport  Port=2
  Demux : Demux  Outputs=2
  Mux : Mux  Inputs=2
  "Sum1 " : Sum  Inputs=+-  SaturateOnIntegerOverflow=on  InputSameDT=on  OutDataTypeStr=Inherit: Same as first input
  Sum2 : Sum  SaturateOnIntegerOverflow=on  InputSameDT=on  OutDataTypeStr=Inherit: Same as first input
  cos : Fcn  Expr=cos(u)
  sin : Fcn  Expr=sin(u)
  x_d*cos : Product  SaturateOnIntegerOverflow=on  RndMeth=Zero  InputSameDT=on  OutDataTypeStr=Inherit: Same as first input
  x_d*sin : Product  SaturateOnIntegerOverflow=on  RndMeth=Zero  InputSameDT=on  OutDataTypeStr=Inherit: Same as first input
  x_q*cos : Product  SaturateOnIntegerOverflow=on  RndMeth=Zero  InputSameDT=on  OutDataTypeStr=Inherit: Same as first input
  "x_q*sin " : Product  SaturateOnIntegerOverflow=on  RndMeth=Zero  InputSameDT=on  OutDataTypeStr=Inherit: Same as first input
  I_ab : Outport
  wires:
  kot/1 -> sin/1, cos/1
  Sum2/1 -> Mux/2
  "Sum1 "/1 -> Mux/1
  x_d*sin/1 -> Sum2/1
  x_q*cos/1 -> Sum2/2
  "x_q*sin "/1 -> "Sum1 "/2
  x_d*cos/1 -> "Sum1 "/1
  sin/1 -> x_d*sin/2, "x_q*sin "/2
  cos/1 -> x_d*cos/2, x_q*cos/2
  Demux/2 -> x_q*cos/1, "x_q*sin "/1
  Demux/1 -> x_d*cos/1, x_d*sin/1
  I_dq/1 -> Demux/1
  Mux/1 -> I_ab/1

== system Model_IPS7/Asinhronski stroj3/Mehanika ==
  M_br : Inport
  M_el : Inport  Port=2
  Sum : Sum  Inputs=+-
  eq 2.19 : Subsystem
  wr : Outport
  wires:
  eq 2.19/1(wr) -> wr/1
  M_el/1 -> Sum/1
  Sum/1 -> eq 2.19/1(M)
  M_br/1 -> Sum/2

== system Model_IPS7/Asinhronski stroj3/Park ==
  U_ab : Inport
  kot : Inport  Port=2
  Demux : Demux  Outputs=2
  Mux : Mux  Inputs=2
  "Sum1 " : Sum  SaturateOnIntegerOverflow=on  InputSameDT=on  OutDataTypeStr=Inherit: Same as first input
  Sum2 : Sum  Inputs=-+  SaturateOnIntegerOverflow=on  InputSameDT=on  OutDataTypeStr=Inherit: Same as first input
  cos : Fcn  Expr=cos(u)
  sin : Fcn  Expr=sin(u)
  x_a*cos : Product  SaturateOnIntegerOverflow=on  RndMeth=Zero  InputSameDT=on  OutDataTypeStr=Inherit: Same as first input
  x_a*sin : Product  SaturateOnIntegerOverflow=on  RndMeth=Zero  InputSameDT=on  OutDataTypeStr=Inherit: Same as first input
  x_b*cos : Product  SaturateOnIntegerOverflow=on  RndMeth=Zero  InputSameDT=on  OutDataTypeStr=Inherit: Same as first input
  "x_b*sin " : Product  SaturateOnIntegerOverflow=on  RndMeth=Zero  InputSameDT=on  OutDataTypeStr=Inherit: Same as first input
  U_dq : Outport
  wires:
  kot/1 -> sin/1, cos/1
  Sum2/1 -> Mux/2
  "Sum1 "/1 -> Mux/1
  x_a*sin/1 -> Sum2/1
  x_b*cos/1 -> Sum2/2
  "x_b*sin "/1 -> "Sum1 "/2
  x_a*cos/1 -> "Sum1 "/1
  sin/1 -> x_a*sin/2, "x_b*sin "/2
  cos/1 -> x_a*cos/2, x_b*cos/2
  Demux/2 -> x_b*cos/1, "x_b*sin "/1
  Demux/1 -> x_a*cos/1, x_a*sin/1
  U_ab/1 -> Demux/1
  Mux/1 -> U_dq/1

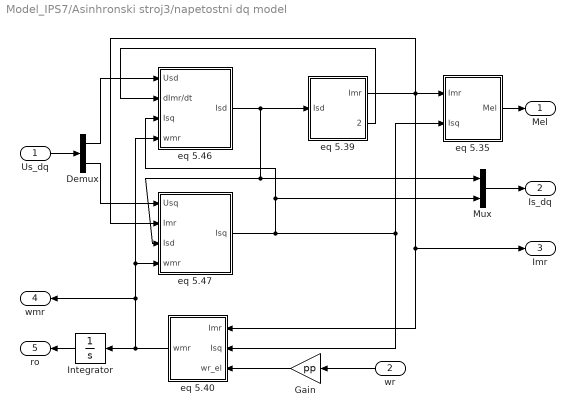
== system Model_IPS7/Asinhronski stroj3/napetostni dq model ==
  Us_dq : Inport
  wr : Inport  Port=2
  Demux : Demux  Outputs=2
  Gain : Gain  Gain=pp
  Integrator : Integrator
  Mux : Mux  Inputs=2
  eq 5.35 : Subsystem
  eq 5.39 : Subsystem
  eq 5.40 : Subsystem
  eq 5.46 : Subsystem
  eq 5.47 : Subsystem
  Mel : Outport
  Is_dq : Outport  Port=2
  Imr : Outport  Port=3
  wmr : Outport  Port=4
  ro : Outport  Port=5
  wires:
  eq 5.46/1(Isd) -> eq 5.39/1(Isd), eq 5.47/3(Isd), Mux/1
  eq 5.39/2(dImr/dt) -> eq 5.46/2(dImr/dt)
  eq 5.39/1(Imr) -> eq 5.35/1(Imr), eq 5.40/1(Imr), Imr/1, eq 5.47/2(Imr)
  eq 5.47/1(Isq) -> eq 5.35/2(Isq), eq 5.40/2(Isq), eq 5.46/3(Isq), Mux/2
  eq 5.40/1(wmr) -> eq 5.47/4(wmr), eq 5.46/4(wmr), wmr/1, Integrator/1
  eq 5.35/1(Mel) -> Mel/1
  Integrator/1 -> ro/1
  wr/1 -> Gain/1
  Us_dq/1 -> Demux/1
  Demux/1 -> eq 5.46/1(Usd)
  Demux/2 -> eq 5.47/1(Usq)
  Mux/1 -> Is_dq/1
  Gain/1 -> eq 5.40/3(wr_el)

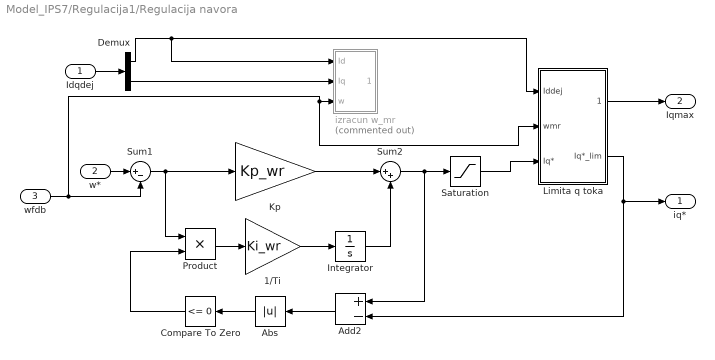
== system Model_IPS7/Regulacija1/Regulacija navora ==
  Idqdej : Inport
  w* : Inport  Port=2
  wfdb : Inport  Port=3
  1/Ti : Gain  Gain=Ki_wr  SaturateOnIntegerOverflow=on  OutDataTypeStr=Inherit: Same as input  ParamDataTypeStr=Inherit: Same as input
  Abs : Abs
  Add2 : Sum  Inputs=+-
  Compare To Zero : simulink/Logic and Bit Operations/Compare To Zero  relop=<=  OutDataTypeStr=boolean
  Demux : Demux  Outputs=2
  Integrator : Integrator
  Kp : Gain  Gain=Kp_wr  SaturateOnIntegerOverflow=on  OutDataTypeStr=Inherit: Same as input  ParamDataTypeStr=Inherit: Same as input
  Limita q toka : Subsystem
  Product : Product
  Saturation : Saturate  UpperLimit=Ismax  LowerLimit=-Ismax
  Sum1 : Sum  Inputs=|+-
  Sum2 : Sum  Inputs=|++
  izracun w_mr : Subsystem  Commented=on
  iq* : Outport
  Iqmax : Outport  Port=2
  wires:
  1/Ti/1 -> Integrator/1
  Sum1/1 -> Product/1, Kp/1
  Integrator/1 -> Sum2/2
  Add2/1 -> Abs/1
  Abs/1 -> Compare To Zero/1
  Kp/1 -> Sum2/1
  Compare To Zero/1 -> Product/2
  Product/1 -> 1/Ti/1
  w*/1 -> Sum1/1
  Sum2/1 -> Saturation/1, Add2/1
  Limita q toka/2(Iq*_lim) -> iq*/1, Add2/2
  Idqdej/1 -> Demux/1
  Limita q toka/1(Iqmaxlim) -> Iqmax/1
  Demux/1 -> izracun w_mr/1(Id), Limita q toka/1(Iddej)
  Saturation/1 -> Limita q toka/3(Iq*)
  Demux/2 -> izracun w_mr/2(Iq)
  wfdb/1 -> Limita q toka/2(wmr), izracun w_mr/3(w), Sum1/2

== system Model_IPS7/Regulacija1/Tok regulator ==
  Idqdej : Inport
  Idq* : Inport  Port=2
  Demux : Demux  Outputs=2
  Demux1 : Demux  Outputs=2
  Dregulator : Subsystem
  Limita Uq : Subsystem
  Mux : Mux  Inputs=2
  Qregulator : Subsystem
  Udq* : Outport
  wires:
  Idq*/1 -> Demux1/1
  Mux/1 -> Udq*/1
  Idqdej/1 -> Demux/1
  Limita Uq/1(Uq_lim) -> Qregulator/3(Uqlim), Mux/2
  Dregulator/1(Ud*(-1:1)) -> Mux/1, Limita Uq/1(Ud)
  Demux1/1 -> Dregulator/1(Id*)
  Demux/1 -> Dregulator/2(Iddej)
  Demux1/2 -> Qregulator/2(Iq*)
  Demux/2 -> Qregulator/1(Iqdej)
  Qregulator/1(Uq*(-1:1)) -> Limita Uq/2(Uq)

== system Model_IPS7/Regulacija1/Transformacije ==
  Udq : Inport
  kot : Inport  Port=2
  I123 : Inport  Port=3
  Clarke : Subsystem
  Inverzni Clarke : Subsystem
  Inverzni Park : Subsystem
  Park : Subsystem
  Idq : Outport
  U123 : Outport  Port=2
  wires:
  Inverzni Clarke/1(U_123) -> U123/1
  Park/1(I_dq) -> Idq/1
  kot/1 -> Inverzni Park/1(kot), Park/2(kot)
  Clarke/1(I_ab) -> Park/1(I_ab)
  Inverzni Park/1(U_ab) -> Inverzni Clarke/1(U_ab)
  Udq/1 -> Inverzni Park/2(U_dq)
  I123/1 -> Clarke/1(I_123)

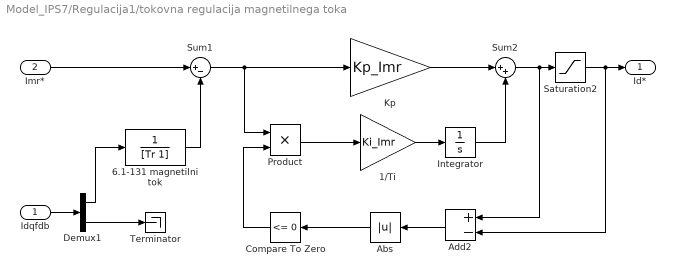
== system Model_IPS7/Regulacija1/tokovna regulacija magnetilnega toka ==
  Idqfdb : Inport
  Imr* : Inport  Port=2
  1/Ti : Gain  Gain=Ki_Imr  SaturateOnIntegerOverflow=on  OutDataTypeStr=Inherit: Same as input  ParamDataTypeStr=Inherit: Same as input
  6.1-131 magnetilni tok : TransferFcn  Denominator=[Tr 1]
  Abs : Abs
  Add2 : Sum  Inputs=+-
  Compare To Zero : simulink/Logic and Bit Operations/Compare To Zero  relop=<=  OutDataTypeStr=boolean
  Demux1 : Demux  Outputs=2
  Integrator : Integrator
  Kp : Gain  Gain=Kp_Imr  SaturateOnIntegerOverflow=on  OutDataTypeStr=Inherit: Same as input  ParamDataTypeStr=Inherit: Same as input
  Product : Product
  Saturation2 : Saturate  UpperLimit=Ismax  LowerLimit=-Ismax
  Sum1 : Sum  Inputs=|+-
  Sum2 : Sum  Inputs=|++
  Terminator : Terminator
  Id* : Outport
  wires:
  Product/1 -> 1/Ti/1
  Compare To Zero/1 -> Product/2
  Abs/1 -> Compare To Zero/1
  Add2/1 -> Abs/1
  Integrator/1 -> Sum2/2
  Imr*/1 -> Sum1/1
  Sum1/1 -> Kp/1, Product/1
  1/Ti/1 -> Integrator/1
  Kp/1 -> Sum2/1
  Demux1/1 -> 6.1-131 magnetilni tok/1
  6.1-131 magnetilni tok/1 -> Sum1/2
  Idqfdb/1 -> Demux1/1
  Sum2/1 -> Add2/1, Saturation2/1
  Saturation2/1 -> Add2/2, Id*/1
  Demux1/2 -> Terminator/1

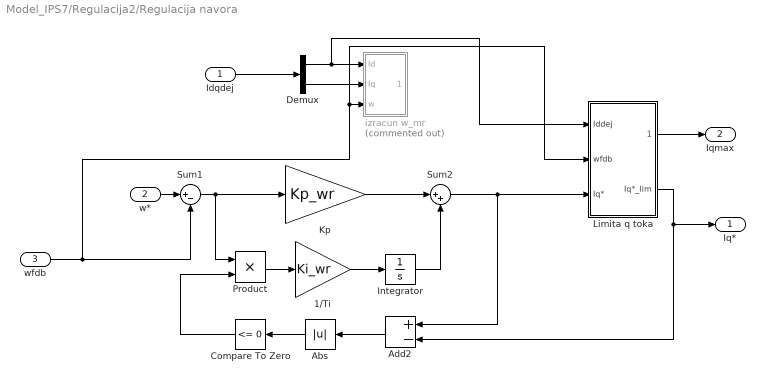
== system Model_IPS7/Regulacija2/Regulacija navora ==
  Idqdej : Inport
  w* : Inport  Port=2
  wfdb : Inport  Port=3
  1/Ti : Gain  Gain=Ki_wr  SaturateOnIntegerOverflow=on  OutDataTypeStr=Inherit: Same as input  ParamDataTypeStr=Inherit: Same as input
  Abs : Abs
  Add2 : Sum  Inputs=+-
  Compare To Zero : simulink/Logic and Bit Operations/Compare To Zero  relop=<=  OutDataTypeStr=boolean
  Demux : Demux  Outputs=2
  Integrator : Integrator
  Kp : Gain  Gain=Kp_wr  SaturateOnIntegerOverflow=on  OutDataTypeStr=Inherit: Same as input  ParamDataTypeStr=Inherit: Same as input
  Limita q toka : Subsystem
  Product : Product
  Sum1 : Sum  Inputs=|+-
  Sum2 : Sum  Inputs=|++
  izracun w_mr : Subsystem  Commented=on
  Iq* : Outport
  Iqmax : Outport  Port=2
  wires:
  1/Ti/1 -> Integrator/1
  Sum1/1 -> Product/1, Kp/1
  Integrator/1 -> Sum2/2
  Add2/1 -> Abs/1
  Abs/1 -> Compare To Zero/1
  Kp/1 -> Sum2/1
  Compare To Zero/1 -> Product/2
  Product/1 -> 1/Ti/1
  w*/1 -> Sum1/1
  Sum2/1 -> Add2/1, Limita q toka/3(Iq*)
  Limita q toka/2(Iq*_lim) -> Iq*/1, Add2/2
  Idqdej/1 -> Demux/1
  Limita q toka/1(Iqmaxlim) -> Iqmax/1
  Demux/1 -> Limita q toka/1(Iddej), izracun w_mr/1(Id)
  Demux/2 -> izracun w_mr/2(Iq)
  wfdb/1 -> Sum1/2, Limita q toka/2(wfdb), izracun w_mr/3(w)

== system Model_IPS7/Regulacija2/Tok regulator ==
  Idqdej : Inport
  Idq* : Inport  Port=2
  Demux : Demux  Outputs=2
  Demux1 : Demux  Outputs=2
  Dregulator : Subsystem
  Limita Uq : Subsystem
  Mux : Mux  Inputs=2
  Qregulator : Subsystem
  Udq* : Outport
  wires:
  Idq*/1 -> Demux1/1
  Mux/1 -> Udq*/1
  Idqdej/1 -> Demux/1
  Limita Uq/1(Uq_lim) -> Qregulator/3(Uqlim), Mux/2
  Dregulator/1(Ud*(-1:1)) -> Mux/1, Limita Uq/1(Ud)
  Demux1/1 -> Dregulator/1(Id*)
  Demux/1 -> Dregulator/2(Iddej)
  Demux1/2 -> Qregulator/2(Iq*)
  Demux/2 -> Qregulator/1(Iqdej)
  Qregulator/1(Uq*(-1:1)) -> Limita Uq/2(Uq)

== system Model_IPS7/Regulacija2/Transformacije ==
  Udq : Inport
  kot : Inport  Port=2
  I123 : Inport  Port=3
  Clarke : Subsystem
  Inverzni Clarke : Subsystem
  Inverzni Park : Subsystem
  Park : Subsystem
  Idq : Outport
  U123 : Outport  Port=2
  wires:
  Inverzni Clarke/1(U_123) -> U123/1
  Park/1(I_dq) -> Idq/1
  kot/1 -> Inverzni Park/1(kot), Park/2(kot)
  Clarke/1(I_ab) -> Park/1(I_ab)
  Inverzni Park/1(U_ab) -> Inverzni Clarke/1(U_ab)
  Udq/1 -> Inverzni Park/2(U_dq)
  I123/1 -> Clarke/1(I_123)

== system Model_IPS7/Regulacija2/tokovna regulacija magnetilnega toka ==
  Idqfdb : Inport
  Imr* : Inport  Port=2
  1/Ti : Gain  Gain=Ki_Imr  SaturateOnIntegerOverflow=on  OutDataTypeStr=Inherit: Same as input  ParamDataTypeStr=Inherit: Same as input
  6.1-131 magnetilni tok : TransferFcn  Denominator=[Tr 1]
  Abs : Abs
  Add2 : Sum  Inputs=+-
  Compare To Zero : simulink/Logic and Bit Operations/Compare To Zero  relop=<=  OutDataTypeStr=boolean
  Demux1 : Demux  Outputs=2
  Integrator : Integrator
  Kp : Gain  Gain=Kp_Imr  SaturateOnIntegerOverflow=on  OutDataTypeStr=Inherit: Same as input  ParamDataTypeStr=Inherit: Same as input
  Product : Product
  Saturation2 : Saturate  UpperLimit=Ismax  LowerLimit=-Ismax
  Sum1 : Sum  Inputs=|+-
  Sum2 : Sum  Inputs=|++
  Terminator : Terminator
  Id* : Outport
  wires:
  Product/1 -> 1/Ti/1
  Compare To Zero/1 -> Product/2
  Abs/1 -> Compare To Zero/1
  Add2/1 -> Abs/1
  Integrator/1 -> Sum2/2
  Imr*/1 -> Sum1/1
  Sum1/1 -> Kp/1, Product/1
  1/Ti/1 -> Integrator/1
  Kp/1 -> Sum2/1
  Demux1/1 -> 6.1-131 magnetilni tok/1
  6.1-131 magnetilni tok/1 -> Sum1/2
  Idqfdb/1 -> Demux1/1
  Sum2/1 -> Add2/1, Saturation2/1
  Saturation2/1 -> Add2/2, Id*/1
  Demux1/2 -> Terminator/1

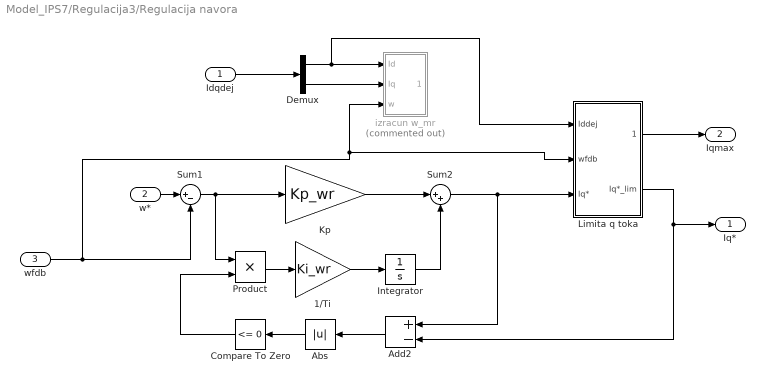
== system Model_IPS7/Regulacija3/Regulacija navora ==
  Idqdej : Inport
  w* : Inport  Port=2
  wfdb : Inport  Port=3
  1/Ti : Gain  Gain=Ki_wr  SaturateOnIntegerOverflow=on  OutDataTypeStr=Inherit: Same as input  ParamDataTypeStr=Inherit: Same as input
  Abs : Abs
  Add2 : Sum  Inputs=+-
  Compare To Zero : simulink/Logic and Bit Operations/Compare To Zero  relop=<=  OutDataTypeStr=boolean
  Demux : Demux  Outputs=2
  Integrator : Integrator
  Kp : Gain  Gain=Kp_wr  SaturateOnIntegerOverflow=on  OutDataTypeStr=Inherit: Same as input  ParamDataTypeStr=Inherit: Same as input
  Limita q toka : Subsystem
  Product : Product
  Sum1 : Sum  Inputs=|+-
  Sum2 : Sum  Inputs=|++
  izracun w_mr : Subsystem  Commented=on
  Iq* : Outport
  Iqmax : Outport  Port=2
  wires:
  wfdb/1 -> Limita q toka/2(wfdb), izracun w_mr/3(w), Sum1/2
  Demux/2 -> izracun w_mr/2(Iq)
  Demux/1 -> izracun w_mr/1(Id), Limita q toka/1(Iddej)
  Limita q toka/1(Iqmaxlim) -> Iqmax/1
  Idqdej/1 -> Demux/1
  Limita q toka/2(Iq*_lim) -> Add2/2, Iq*/1
  Sum2/1 -> Limita q toka/3(Iq*), Add2/1
  w*/1 -> Sum1/1
  Product/1 -> 1/Ti/1
  Compare To Zero/1 -> Product/2
  Kp/1 -> Sum2/1
  Abs/1 -> Compare To Zero/1
  Add2/1 -> Abs/1
  Integrator/1 -> Sum2/2
  Sum1/1 -> Kp/1, Product/1
  1/Ti/1 -> Integrator/1

== system Model_IPS7/Regulacija3/Tok regulator ==
  Idqdej : Inport
  Idq* : Inport  Port=2
  Demux : Demux  Outputs=2
  Demux1 : Demux  Outputs=2
  Dregulator : Subsystem
  Limita Uq : Subsystem
  Mux : Mux  Inputs=2
  Qregulator : Subsystem
  Udq* : Outport
  wires:
  Qregulator/1(Uq*(-1:1)) -> Limita Uq/2(Uq)
  Demux/1 -> Dregulator/2(Iddej)
  Demux1/1 -> Dregulator/1(Id*)
  Dregulator/1(Ud*(-1:1)) -> Limita Uq/1(Ud), Mux/1
  Limita Uq/1(Uq_lim) -> Mux/2, Qregulator/3(Uqlim)
  Idqdej/1 -> Demux/1
  Mux/1 -> Udq*/1
  Idq*/1 -> Demux1/1
  Demux/2 -> Qregulator/1(Iqdej)
  Demux1/2 -> Qregulator/2(Iq*)

== system Model_IPS7/Regulacija3/Transformacije ==
  Udq : Inport
  kot : Inport  Port=2
  I123 : Inport  Port=3
  Clarke : Subsystem
  Inverzni Clarke : Subsystem
  Inverzni Park : Subsystem
  Park : Subsystem
  Idq : Outport
  U123 : Outport  Port=2
  wires:
  I123/1 -> Clarke/1(I_123)
  Udq/1 -> Inverzni Park/2(U_dq)
  Inverzni Park/1(U_ab) -> Inverzni Clarke/1(U_ab)
  Clarke/1(I_ab) -> Park/1(I_ab)
  kot/1 -> Park/2(kot), Inverzni Park/1(kot)
  Park/1(I_dq) -> Idq/1
  Inverzni Clarke/1(U_123) -> U123/1

== system Model_IPS7/Regulacija3/tokovna regulacija magnetilnega toka ==
  Idqfdb : Inport
  Imr* : Inport  Port=2
  1/Ti : Gain  Gain=Ki_Imr  SaturateOnIntegerOverflow=on  OutDataTypeStr=Inherit: Same as input  ParamDataTypeStr=Inherit: Same as input
  6.1-131 magnetilni tok : TransferFcn  Denominator=[Tr 1]
  Abs : Abs
  Add2 : Sum  Inputs=+-
  Compare To Zero : simulink/Logic and Bit Operations/Compare To Zero  relop=<=  OutDataTypeStr=boolean
  Demux1 : Demux  Outputs=2
  Integrator : Integrator
  Kp : Gain  Gain=Kp_Imr  SaturateOnIntegerOverflow=on  OutDataTypeStr=Inherit: Same as input  ParamDataTypeStr=Inherit: Same as input
  Product : Product
  Saturation2 : Saturate  UpperLimit=Ismax  LowerLimit=-Ismax
  Sum1 : Sum  Inputs=|+-
  Sum2 : Sum  Inputs=|++
  Terminator : Terminator
  Id* : Outport
  wires:
  Demux1/2 -> Terminator/1
  Saturation2/1 -> Id*/1, Add2/2
  Sum2/1 -> Saturation2/1, Add2/1
  Idqfdb/1 -> Demux1/1
  6.1-131 magnetilni tok/1 -> Sum1/2
  Demux1/1 -> 6.1-131 magnetilni tok/1
  Kp/1 -> Sum2/1
  1/Ti/1 -> Integrator/1
  Sum1/1 -> Product/1, Kp/1
  Imr*/1 -> Sum1/1
  Integrator/1 -> Sum2/2
  Add2/1 -> Abs/1
  Abs/1 -> Compare To Zero/1
  Compare To Zero/1 -> Product/2
  Product/1 -> 1/Ti/1

== system Model_IPS7/TechniqueB1/Const c ==
  Id : Inport
  6.1-1 : TransferFcn  Numerator=[-Tr*Lm^2/Lr 0]  Denominator=[Tr 1]
  6.1-2 : TransferFcn  Denominator=[1 1]
  c : Outport
  wires:
  Id/1 -> 6.1-1/1
  6.1-1/1 -> 6.1-2/1
  6.1-2/1 -> c/1

== system Model_IPS7/TechniqueB1/Korenski del ==
  c : Inport
  w : Inport  Port=2
  Add1 : Sum  Inputs=--+
  Add2 : Sum
  Add3 : Sum
  Constant1 : Constant  Value=Udc
  Constant2 : Constant  Value=0.000001
  Constant3 : Constant  Value=Lst^2*Ismax^2
  Divide : Product  Inputs=*/
  Gain3 : Gain  Gain=Ls^2-Lst^2
  Gain5 : Gain  Gain=Ls^2
  Product3 : Product
  Product4 : Product
  Saturation1 : Saturate  UpperLimit=wb_upper_limit_field_weaking  LowerLimit=-wb_upper_limit_field_weaking
  Sqrt : Sqrt  SaturateOnIntegerOverflow=on
  korenjen del : Outport
  wires:
  c/1 -> Product4/2, Product4/1
  Product4/1 -> Add1/1, Gain5/1
  Saturation1/1 -> Add2/1
  Constant1/1 -> Divide/1
  Constant2/1 -> Add2/2
  Add1/1 -> Gain3/1
  Add2/1 -> Divide/2
  w/1 -> Saturation1/1
  Divide/1 -> Product3/1, Product3/2
  Product3/1 -> Add1/3
  Sqrt/1 -> korenjen del/1
  Add3/1 -> Sqrt/1
  Gain5/1 -> Add3/1
  Gain3/1 -> Add3/2
  Constant3/1 -> Add1/2

== system Model_IPS7/Time&random/99% max navora ==
  "\tIdq" : Inport
  Iqmax : Inport  Port=2
  Demux : Demux  Outputs=2
  Gain1 : Gain  Gain=3*pp/2
  Gain2 : Gain  Gain=Lm*Lm/Lr
  Product2 : Product  Inputs=3  RndMeth=Zero
  Step : Step  Time=0.6  After=0.99  SampleTime=0
  Out1 : Outport
  wires:
  "\tIdq"/1 -> Demux/1
  Demux/1 -> Product2/1
  Iqmax/1 -> Product2/2
  Step/1 -> Product2/3
  Gain1/1 -> Gain2/1
  Product2/1 -> Gain1/1
  Gain2/1 -> Out1/1

== system Model_IPS7/Asinhronski stroj1/Clarke/ABC_ab1 ==
  A : Inport
  B : Inport  Port=2
  C : Inport  Port=3
  Gain1 : Gain  Gain=2
  Gain2 : Gain
  Gain24 : Gain  Gain=sqrt(3)/3
  Sum11 : Sum
  Terminator : Terminator
  alfa : Outport
  beta : Outport  Port=2
  wires:
  C/1 -> Terminator/1
  Gain1/1 -> Sum11/2
  B/1 -> Gain1/1
  Gain24/1 -> beta/1
  Gain2/1 -> alfa/1
  Sum11/1 -> Gain24/1
  A/1 -> Sum11/1, Gain2/1

== system Model_IPS7/Asinhronski stroj1/Inverzni Clarke/ab_ABC ==
  alfa : Inport
  beta : Inport  Port=2
  Gain1 : Gain
  Gain2 : Gain  Gain=-0.5
  Gain25 : Gain  Gain=sqrt(3)/2
  Gain3 : Gain  Gain=sqrt(3)/2
  Gain4 : Gain  Gain=0.5
  Sum10 : Sum
  Sum11 : Sum  Inputs=--
  A : Outport
  B : Outport  Port=2
  C : Outport  Port=3
  wires:
  Gain3/1 -> Sum11/2
  beta/1 -> Gain25/1, Gain3/1
  Gain4/1 -> Sum11/1
  Gain25/1 -> Sum10/2
  Gain2/1 -> Sum10/1
  alfa/1 -> Gain1/1, Gain2/1, Gain4/1
  Gain1/1 -> A/1
  Sum10/1 -> B/1
  Sum11/1 -> C/1

== system Model_IPS7/Asinhronski stroj1/Mehanika/eq 2.19 ==
  M : Inport
  Gain1 : Gain  Gain=1/J
  Integrator : Integrator
  wr : Outport
  wires:
  Integrator/1 -> wr/1
  M/1 -> Gain1/1
  Gain1/1 -> Integrator/1

== system Model_IPS7/Asinhronski stroj1/napetostni dq model/eq 5.35 ==
  Imr : Inport
  Isq : Inport  Port=2
  Gain : Gain  Gain=3*pp/2
  Gain2 : Gain  Gain=Lm*Lm/Lr
  Product : Product  RndMeth=Zero
  Mel : Outport
  wires:
  Gain/1 -> Gain2/1
  Gain2/1 -> Mel/1
  Product/1 -> Gain/1
  Isq/1 -> Product/2
  Imr/1 -> Product/1

== system Model_IPS7/Asinhronski stroj1/napetostni dq model/eq 5.39 ==
  Isd : Inport
  Gain : Gain  Gain=1/Tr
  Integrator : Integrator  InitialCondition=1e-3
  Sum : Sum  Inputs=|+-
  Imr : Outport
  dImr/dt : Outport  Port=2
  wires:
  Gain/1 -> dImr/dt/1, Integrator/1
  Sum/1 -> Gain/1
  Integrator/1 -> Sum/2, Imr/1
  Isd/1 -> Sum/1

== system Model_IPS7/Asinhronski stroj1/napetostni dq model/eq 5.40 ==
  Imr : Inport
  Isq : Inport  Port=2
  wr_el : Inport  Port=3
  Divide : Product  Inputs=*/
  Gain2 : Gain  Gain=Tr
  Saturation : Saturate  UpperLimit=2*pi*50  LowerLimit=-2*pi*50
  Sum : Sum  Inputs=|++
  wmr : Outport
  wires:
  Saturation/1 -> Sum/1
  Sum/1 -> wmr/1
  wr_el/1 -> Sum/2
  Divide/1 -> Saturation/1  "ws"
  Gain2/1 -> Divide/2
  Imr/1 -> Gain2/1
  Isq/1 -> Divide/1

== system Model_IPS7/Asinhronski stroj1/napetostni dq model/eq 5.46 ==
  Usd : Inport
  dImr/dt : Inport  Port=2
  Isq : Inport  Port=3
  wmr : Inport  Port=4
  Gain : Gain  Gain=1/(sigma*Ls)
  Gain1 : Gain  Gain=Rs
  Gain2 : Gain  Gain=(1-sigma)*Ls
  Gain3 : Gain  Gain=sigma*Ls
  Integrator : Integrator
  Product : Product  RndMeth=Zero
  Sum : Sum  Inputs=+--+
  Isd : Outport
  wires:
  Gain3/1 -> Sum/4
  Product/1 -> Gain3/1
  Isq/1 -> Product/1
  wmr/1 -> Product/2
  Gain2/1 -> Sum/3
  dImr/dt/1 -> Gain2/1
  Gain1/1 -> Sum/2
  Usd/1 -> Sum/1
  Sum/1 -> Gain/1
  Gain/1 -> Integrator/1
  Integrator/1 -> Gain1/1, Isd/1

== system Model_IPS7/Asinhronski stroj1/napetostni dq model/eq 5.47 ==
  Usq : Inport
  Imr : Inport  Port=2
  Isd : Inport  Port=3
  wmr : Inport  Port=4
  Gain : Gain  Gain=1/(sigma*Ls)
  Gain1 : Gain  Gain=Rs
  Gain2 : Gain  Gain=(1-sigma)*Ls
  Gain3 : Gain  Gain=sigma*Ls
  Integrator : Integrator
  Product : Product  RndMeth=Zero
  Product1 : Product  RndMeth=Zero
  Sum : Sum  Inputs=+---
  Isq : Outport
  wires:
  Gain3/1 -> Sum/4
  Product1/1 -> Gain3/1
  Isd/1 -> Product1/2
  Gain2/1 -> Sum/3
  Product/1 -> Gain2/1
  wmr/1 -> Product1/1, Product/2
  Imr/1 -> Product/1
  Gain1/1 -> Sum/2
  Usq/1 -> Sum/1
  Sum/1 -> Gain/1
  Gain/1 -> Integrator/1
  Integrator/1 -> Gain1/1, Isq/1

== system Model_IPS7/Asinhronski stroj2/Clarke/ABC_ab1 ==
  A : Inport
  B : Inport  Port=2
  C : Inport  Port=3
  Gain1 : Gain  Gain=2
  Gain2 : Gain
  Gain24 : Gain  Gain=sqrt(3)/3
  Sum11 : Sum
  Terminator : Terminator
  alfa : Outport
  beta : Outport  Port=2
  wires:
  C/1 -> Terminator/1
  Gain1/1 -> Sum11/2
  B/1 -> Gain1/1
  Gain24/1 -> beta/1
  Gain2/1 -> alfa/1
  Sum11/1 -> Gain24/1
  A/1 -> Sum11/1, Gain2/1

== system Model_IPS7/Asinhronski stroj2/Inverzni Clarke/ab_ABC ==
  alfa : Inport
  beta : Inport  Port=2
  Gain1 : Gain
  Gain2 : Gain  Gain=-0.5
  Gain25 : Gain  Gain=sqrt(3)/2
  Gain3 : Gain  Gain=sqrt(3)/2
  Gain4 : Gain  Gain=0.5
  Sum10 : Sum
  Sum11 : Sum  Inputs=--
  A : Outport
  B : Outport  Port=2
  C : Outport  Port=3
  wires:
  Gain3/1 -> Sum11/2
  beta/1 -> Gain25/1, Gain3/1
  Gain4/1 -> Sum11/1
  Gain25/1 -> Sum10/2
  Gain2/1 -> Sum10/1
  alfa/1 -> Gain1/1, Gain2/1, Gain4/1
  Gain1/1 -> A/1
  Sum10/1 -> B/1
  Sum11/1 -> C/1

== system Model_IPS7/Asinhronski stroj2/Mehanika/eq 2.19 ==
  M : Inport
  Gain1 : Gain  Gain=1/J
  Integrator : Integrator
  wr : Outport
  wires:
  Integrator/1 -> wr/1
  M/1 -> Gain1/1
  Gain1/1 -> Integrator/1

== system Model_IPS7/Asinhronski stroj2/napetostni dq model/eq 5.35 ==
  Imr : Inport
  Isq : Inport  Port=2
  Gain : Gain  Gain=3*pp/2
  Gain2 : Gain  Gain=Lm*Lm/Lr
  Product : Product  RndMeth=Zero
  Mel : Outport
  wires:
  Gain/1 -> Gain2/1
  Gain2/1 -> Mel/1
  Product/1 -> Gain/1
  Isq/1 -> Product/2
  Imr/1 -> Product/1

== system Model_IPS7/Asinhronski stroj2/napetostni dq model/eq 5.39 ==
  Isd : Inport
  Gain : Gain  Gain=1/Tr
  Integrator : Integrator  InitialCondition=1e-3
  Sum : Sum  Inputs=|+-
  Imr : Outport
  dImr/dt : Outport  Port=2
  wires:
  Gain/1 -> dImr/dt/1, Integrator/1
  Sum/1 -> Gain/1
  Integrator/1 -> Sum/2, Imr/1
  Isd/1 -> Sum/1

== system Model_IPS7/Asinhronski stroj2/napetostni dq model/eq 5.40 ==
  Imr : Inport
  Isq : Inport  Port=2
  wr_el : Inport  Port=3
  Divide : Product  Inputs=*/
  Gain2 : Gain  Gain=Tr
  Saturation : Saturate  UpperLimit=2*pi*50  LowerLimit=-2*pi*50
  Sum : Sum  Inputs=|++
  wmr : Outport
  wires:
  Saturation/1 -> Sum/1
  Sum/1 -> wmr/1
  wr_el/1 -> Sum/2
  Divide/1 -> Saturation/1  "ws"
  Gain2/1 -> Divide/2
  Imr/1 -> Gain2/1
  Isq/1 -> Divide/1
